simulink model "LA3"  (R2020a)
settings: Solver=VariableStepAuto  StartTime=0.0  StopTime=10.0  RelTol=1e-3
libraries: Regler x6
settings Model: Creator=Admin  LastModifiedBy=bradfisch

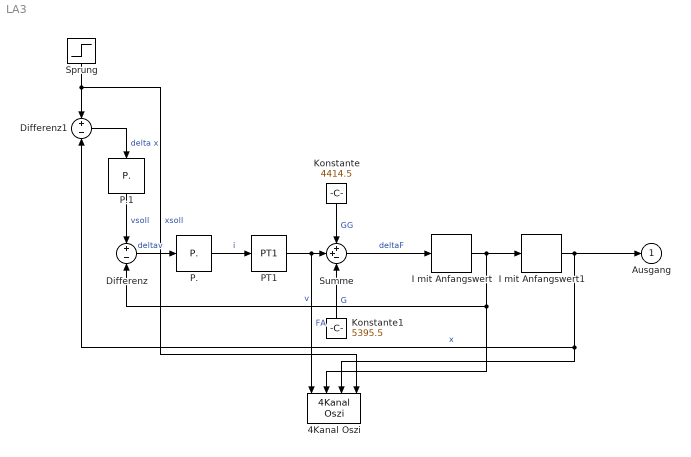
== system LA3 ==
  4Kanal Oszi : Regler/4Kanal Oszi  N=20000  k=[1/100 1 1 1/20]  y=[-5 5]  tmax=1
  Differenz : Sum  Inputs=+-  InputSameDT=on  SaturateOnIntegerOverflow=on  OutDataTypeStr=Inherit: Same as first input
  Differenz1 : Sum  Inputs=+-  InputSameDT=on  SaturateOnIntegerOverflow=on  OutDataTypeStr=Inherit: Same as first input
  I mit Anfangswert : Regler/I mit Anfangswert  Ti=550+450  u0=0
  I mit Anfangswert1 : Regler/I mit Anfangswert  Ti=1  u0=10
  Konstante : Constant  Value=4414.5
  Konstante1 : Constant  Value=5395.5
  P. : Regler/P.  k=25
  P.1 : Regler/P.  k=4
  PT1 : Regler/PT1  k=100  T1=0.2
  Sprung : Step  Time=0.000001  Before=10  After=16  SampleTime=0
  Summe : Sum  Inputs=++-  InputSameDT=on  SaturateOnIntegerOverflow=on  OutDataTypeStr=Inherit: Same as first input
  Ausgang : Outport  VectorParamsAs1DForOutWhenUnconnected=off
  wires:
  P./1 -> PT1/1  "i"
  I mit Anfangswert/1 -> Differenz/2, 4Kanal Oszi/2, I mit Anfangswert1/1  "v"
  I mit Anfangswert1/1 -> Differenz1/2, 4Kanal Oszi/3, Ausgang/1  "x"
  Konstante/1 -> Summe/1  "GG"
  PT1/1 -> 4Kanal Oszi/1, Summe/2  "FA"
  Konstante1/1 -> Summe/3  "G"
  Summe/1 -> I mit Anfangswert/1  "deltaF"
  Sprung/1 -> 4Kanal Oszi/4, Differenz1/1  "xsoll"
  Differenz/1 -> P./1  "deltav"
  P.1/1 -> Differenz/1  "vsoll"
  Differenz1/1 -> P.1/1  "delta x"
